simulink model "Pacemaker"  (R2023a)
settings: Solver=FixedStepAuto  StartTime=0.0  StopTime=inf  FixedStep=0.001  RelTol=1e-3  EnableMultiTasking=on
undefined symbols (not defined in the file): D0, D1, D10, D11, D12, D13, D2, D3, D4, D5, D6, D7, D8, D9, PTA0, PTA1, PTA2, PTB23, PTB9, PTC16, PTC17, PTC2, PTC3, PTC4, PTD0, PTD1, PTD2, PTD3
libraries: frdmk64flib x15
settings Model: ExtModeTrigDuration=5  Creator=tstic  LastModifiedBy=nehac
settings OptimizationCC: EnhancedBackFolding=on  PassReuseOutputArgsAs=Individual arguments  ZeroExternalMemoryAtStartup=off  ZeroInternalMemoryAtStartup=off  MaxStackSize=64  OptimizeBlockOrder=speed  DifferentSizesBufferReuse=on  OptimizationCustomize=off  EfficientTunableParamExpr=on
settings DebuggingCC: ParameterTunabilityLossMsg=error
settings HardwareCC: ProdBitPerPointer=32  ProdBitPerSizeT=32  ProdBitPerPtrDiffT=32  ProdLargestAtomicInteger=Long  ProdLargestAtomicFloat=Double  ProdWordSize=32  ProdHWDeviceType=ARM Compatible->ARM Cortex
settings SFSimCC: MATLABDynamicMemAlloc=off
settings RTWCC: Description=Embedded Coder  SystemTargetFile=ert.tlc  HardwareBoard=NXP FRDM-K64F  TLCOptions="-aInlineSetEventsForThisBaseRateFcn=TLC_FALSE -aSuppressMultiTaskScheduler=TLC_FALSE  -aRateBasedStepFcn=0"  TemplateMakefile=ert_default_tmf  Toolchain=GNU Tools for ARM Embedded Processors
settings CodeAppCC: ForceParamTrailComments=on  IgnoreCustomStorageClasses=off  OperatorAnnotations=on  SimulinkDataObjDesc=on  SFDataObjDesc=on  InsertBlockDesc=on
settings ERTTargetCC: ExtModeTransport=4  ExtModeMexFile=sendToCommService

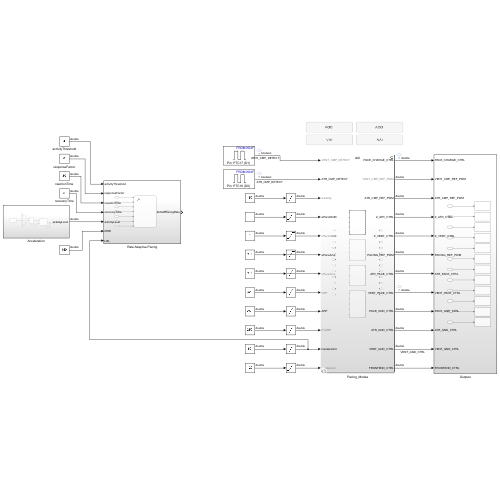
[thumbnail: Simulink's stored preview of the top-level diagram]
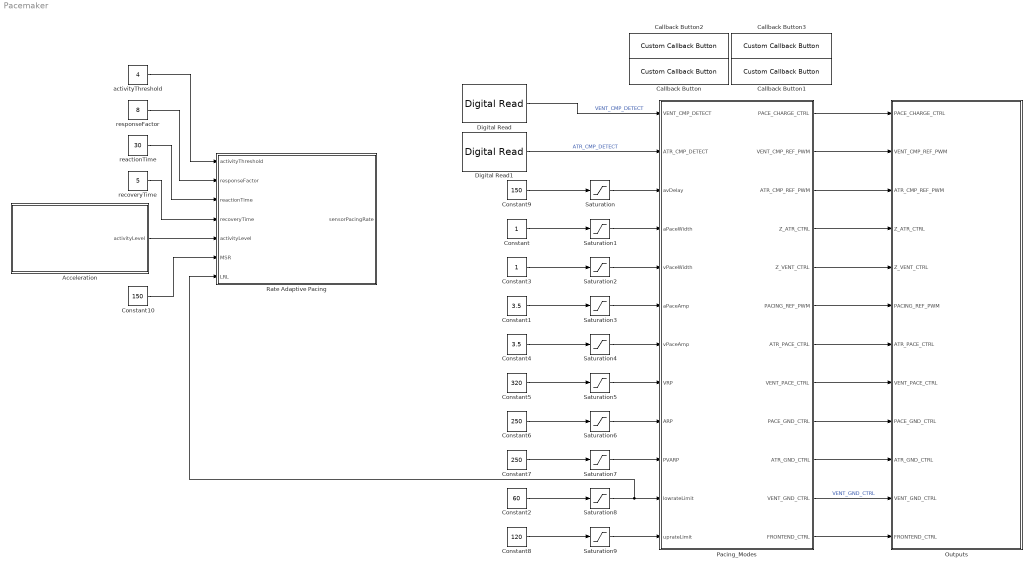
== system Pacemaker ==
  Acceleration : Subsystem
  Callback Button : CustomCallbackButton  Configuration="{\"components\":[{\"name\":\"BackgroundImageComponent\",\"settings\":{\"image\":{\"size\":[0,0],\"src\":\"default\",\"srcOrientation\":\"Right\"},\"position\":[0,0,1,1]}},{\"name\":\"ButtonStateComponent\",\"settings\":{\"buttonType\":\"momentary\",\"clickFcn\":\"myVCV = PacingMode.VVI;\",\"onValue\":1,\"position\":[0,0,1,1],\"pressDelay\":\"500\",\"pressFcn\":\"\",\"repeatInterval\":\"0\",\"states\":[{\"horizontalAlignment\":\"center\",\"image\":{\"position\":[0,0,1,1],\"size\":[1,1],\"src\":\"default\",\"srcOrientation\":\"Right\"},\"label\":{\"color\":[0.01176470588,0.01176470588,0.01176470588,1],\"icon\":{\"size\":[0,0],\"src\":\"default\",\"srcOrientation\":\"Right\"},\"iconPlacement\":\"left\",\"opacity\":1,\"show\":true,\"text\":{\"content\":\"VVI\",\"font\":\"Helvetica\",\"fontSize\":24}},\"labelOffset\":[0,0],\"verticalAlignment\":\"middle\"},{\"horizontalAlignment\":\"center\",\"image\":{\"position\":[0,0,1,1],\"size\":[1,1],\"src\":\"default\",\"srcOrientation\":\"Right\"},\"label\":{\"color\":[0.01176470588,0.01176470588,0.01176470588,1],\"icon\":{\"size\":[0,0],\"src\":\"default\",\"srcOrientation\":\"Right\"},\"iconPlacement\":\"left\",\"opacity\":1,\"show\":true,\"text\":{\"content\":\"VVI\",\"font\":\"Helvetica\",\"fontSize\":24}},\"labelOffset\":[0,0],\"verticalAlignment\":\"middle\"},{\"horizontalAlignment\":\"center\",\"image\":{\"position\":[0,0,1,1],\"size\":[1,1],\"src\":\"default\",\"srcOrientation\":\"Right\"},\"label\":{\"color\":[0.01176470588,0.01176470588,0.01176470588,1],\"icon\":{\"size\":[0,0],\"src\":\"default\",\"srcOrientation\":\"Right\"},\"iconPlacement\":\"left\",\"opacity\":1,\"show\":true,\"text\":{\"content\":\"VVI\",\"font\":\"Helvetica\",\"fontSize\":24}},\"labelOffset\":[0,0],\"verticalAlignment\":\"middle\"},{\"horizontalAlignment\":\"center\",\"image\":{\"position\":[0,0,1,1],\"size\":[1,1],\"src\":\"default\",\"srcOrientation\":\"Right\"},\"label\":{\"color\":[0.01176470588,0.01176470588,0.01176470588,1],\"icon\":{\"size\":[0,0],\"src\":\"default\",\"srcOrientation\":\"Right\"},\"iconPlacement\":\"left\",\"opacity\":1,\"show\":true,\"text\":{\"content\":\"VVI\",\"font\":\"Helvetica\",\"fontSize\":24}},\"labelOffset\":[0,0],\"verticalAlignment\":\"middle\"}]}},{\"name\":\"ForegroundImageComponent\",\"settings\":{\"image\":{\"size\":[0,0],\"src\":\"default\",\"srcOrientation\":\"Right\"},\"isForeground\":1,\"position\":[0,0,1,1]}}],\"settings\":{\"BindingType\":\"standalone\",\"backgroundColor\":[244,244,244,1],\"backgroundOffset\":0.2,\"backgroundOpacity\":1,\"fixedAspectRatio\":\"off\",\"foregroundColor\":[0.01176470588,0.01176470588,0.01176470588,1],\"migratedFromLegacy\":true,\"useBackgroundColor\":true,\"variant\":\"callback\",\"version\":\"R2023a\"},\"type\":\"Button\"}"  CustomBackgroundColor="{\"color\":[0.9568627450980393,0.9568627450980393,0.9568627450980393],\"show\":true}"
  Callback Button1 : CustomCallbackButton  Configuration="{\"components\":[{\"name\":\"BackgroundImageComponent\",\"settings\":{\"image\":{\"size\":[0,0],\"src\":\"default\",\"srcOrientation\":\"Right\"},\"position\":[0,0,1,1]}},{\"name\":\"ButtonStateComponent\",\"settings\":{\"buttonType\":\"momentary\",\"clickFcn\":\"myVCV = PacingMode.AAI;\",\"onValue\":1,\"position\":[0,0,1,1],\"pressDelay\":\"500\",\"pressFcn\":\"\",\"repeatInterval\":\"0\",\"states\":[{\"horizontalAlignment\":\"center\",\"image\":{\"position\":[0,0,1,1],\"size\":[1,1],\"src\":\"default\",\"srcOrientation\":\"Right\"},\"label\":{\"color\":[0.01176470588,0.01176470588,0.01176470588,1],\"icon\":{\"size\":[0,0],\"src\":\"default\",\"srcOrientation\":\"Right\"},\"iconPlacement\":\"left\",\"opacity\":1,\"show\":true,\"text\":{\"content\":\"AAI\",\"font\":\"Helvetica\",\"fontSize\":27}},\"labelOffset\":[0,0],\"verticalAlignment\":\"middle\"},{\"horizontalAlignment\":\"center\",\"image\":{\"position\":[0,0,1,1],\"size\":[1,1],\"src\":\"default\",\"srcOrientation\":\"Right\"},\"label\":{\"color\":[0.01176470588,0.01176470588,0.01176470588,1],\"icon\":{\"size\":[0,0],\"src\":\"default\",\"srcOrientation\":\"Right\"},\"iconPlacement\":\"left\",\"opacity\":1,\"show\":true,\"text\":{\"content\":\"AAI\",\"font\":\"Helvetica\",\"fontSize\":27}},\"labelOffset\":[0,0],\"verticalAlignment\":\"middle\"},{\"horizontalAlignment\":\"center\",\"image\":{\"position\":[0,0,1,1],\"size\":[1,1],\"src\":\"default\",\"srcOrientation\":\"Right\"},\"label\":{\"color\":[0.01176470588,0.01176470588,0.01176470588,1],\"icon\":{\"size\":[0,0],\"src\":\"default\",\"srcOrientation\":\"Right\"},\"iconPlacement\":\"left\",\"opacity\":1,\"show\":true,\"text\":{\"content\":\"AAI\",\"font\":\"Helvetica\",\"fontSize\":27}},\"labelOffset\":[0,0],\"verticalAlignment\":\"middle\"},{\"horizontalAlignment\":\"center\",\"image\":{\"position\":[0,0,1,1],\"size\":[1,1],\"src\":\"default\",\"srcOrientation\":\"Right\"},\"label\":{\"color\":[0.01176470588,0.01176470588,0.01176470588,1],\"icon\":{\"size\":[0,0],\"src\":\"default\",\"srcOrientation\":\"Right\"},\"iconPlacement\":\"left\",\"opacity\":1,\"show\":true,\"text\":{\"content\":\"AAI\",\"font\":\"Helvetica\",\"fontSize\":27}},\"labelOffset\":[0,0],\"verticalAlignment\":\"middle\"}]}},{\"name\":\"ForegroundImageComponent\",\"settings\":{\"image\":{\"size\":[0,0],\"src\":\"default\",\"srcOrientation\":\"Right\"},\"isForeground\":1,\"position\":[0,0,1,1]}}],\"settings\":{\"BindingType\":\"standalone\",\"backgroundColor\":[244,244,244,1],\"backgroundOffset\":0.2,\"backgroundOpacity\":1,\"fixedAspectRatio\":\"off\",\"foregroundColor\":[0.01176470588,0.01176470588,0.01176470588,1],\"migratedFromLegacy\":true,\"useBackgroundColor\":true,\"variant\":\"callback\",\"version\":\"R2023a\"},\"type\":\"Button\"}"  CustomBackgroundColor="{\"color\":[0.9568627450980393,0.9568627450980393,0.9568627450980393],\"show\":true}"
  Callback Button2 : CustomCallbackButton  Configuration="{\"components\":[{\"name\":\"BackgroundImageComponent\",\"settings\":{\"image\":{\"size\":[0,0],\"src\":\"default\",\"srcOrientation\":\"Right\"},\"position\":[0,0,1,1]}},{\"name\":\"ButtonStateComponent\",\"settings\":{\"buttonType\":\"momentary\",\"clickFcn\":\"myVCV = PacingMode.VOO;\",\"onValue\":1,\"position\":[0,0,1,1],\"pressDelay\":\"500\",\"pressFcn\":\"\",\"repeatInterval\":\"0\",\"states\":[{\"horizontalAlignment\":\"center\",\"image\":{\"position\":[0,0,1,1],\"size\":[1,1],\"src\":\"default\",\"srcOrientation\":\"Right\"},\"label\":{\"color\":[0.01176470588,0.01176470588,0.01176470588,1],\"icon\":{\"size\":[0,0],\"src\":\"default\",\"srcOrientation\":\"Right\"},\"iconPlacement\":\"left\",\"opacity\":1,\"show\":true,\"text\":{\"content\":\"VOO\",\"font\":\"Helvetica\",\"fontSize\":27}},\"labelOffset\":[0,0],\"verticalAlignment\":\"middle\"},{\"horizontalAlignment\":\"center\",\"image\":{\"position\":[0,0,1,1],\"size\":[1,1],\"src\":\"default\",\"srcOrientation\":\"Right\"},\"label\":{\"color\":[0.01176470588,0.01176470588,0.01176470588,1],\"icon\":{\"size\":[0,0],\"src\":\"default\",\"srcOrientation\":\"Right\"},\"iconPlacement\":\"left\",\"opacity\":1,\"show\":true,\"text\":{\"content\":\"VOO\",\"font\":\"Helvetica\",\"fontSize\":27}},\"labelOffset\":[0,0],\"verticalAlignment\":\"middle\"},{\"horizontalAlignment\":\"center\",\"image\":{\"position\":[0,0,1,1],\"size\":[1,1],\"src\":\"default\",\"srcOrientation\":\"Right\"},\"label\":{\"color\":[0.01176470588,0.01176470588,0.01176470588,1],\"icon\":{\"size\":[0,0],\"src\":\"default\",\"srcOrientation\":\"Right\"},\"iconPlacement\":\"left\",\"opacity\":1,\"show\":true,\"text\":{\"content\":\"VOO\",\"font\":\"Helvetica\",\"fontSize\":27}},\"labelOffset\":[0,0],\"verticalAlignment\":\"middle\"},{\"horizontalAlignment\":\"center\",\"image\":{\"position\":[0,0,1,1],\"size\":[1,1],\"src\":\"default\",\"srcOrientation\":\"Right\"},\"label\":{\"color\":[0.01176470588,0.01176470588,0.01176470588,1],\"icon\":{\"size\":[0,0],\"src\":\"default\",\"srcOrientation\":\"Right\"},\"iconPlacement\":\"left\",\"opacity\":1,\"show\":true,\"text\":{\"content\":\"VOO\",\"font\":\"Helvetica\",\"fontSize\":27}},\"labelOffset\":[0,0],\"verticalAlignment\":\"middle\"}]}},{\"name\":\"ForegroundImageComponent\",\"settings\":{\"image\":{\"size\":[0,0],\"src\":\"default\",\"srcOrientation\":\"Right\"},\"isForeground\":1,\"position\":[0,0,1,1]}}],\"settings\":{\"BindingType\":\"standalone\",\"backgroundColor\":[244,244,244,1],\"backgroundOffset\":0.2,\"backgroundOpacity\":1,\"fixedAspectRatio\":\"off\",\"foregroundColor\":[0.01176470588,0.01176470588,0.01176470588,1],\"migratedFromLegacy\":true,\"useBackgroundColor\":true,\"variant\":\"callback\",\"version\":\"R2023a\"},\"type\":\"Button\"}"  CustomBackgroundColor="{\"color\":[0.9568627450980393,0.9568627450980393,0.9568627450980393],\"show\":true}"
  Callback Button3 : CustomCallbackButton  Configuration="{\"components\":[{\"name\":\"BackgroundImageComponent\",\"settings\":{\"image\":{\"size\":[0,0],\"src\":\"default\",\"srcOrientation\":\"Right\"},\"position\":[0,0,1,1]}},{\"name\":\"ButtonStateComponent\",\"settings\":{\"buttonType\":\"momentary\",\"clickFcn\":\"myVCV = PacingMode.AOO;\",\"onValue\":1,\"position\":[0,0,1,1],\"pressDelay\":\"500\",\"pressFcn\":\"\",\"repeatInterval\":\"0\",\"states\":[{\"horizontalAlignment\":\"center\",\"image\":{\"position\":[0,0,1,1],\"size\":[1,1],\"src\":\"default\",\"srcOrientation\":\"Right\"},\"label\":{\"color\":[0.01176470588,0.01176470588,0.01176470588,1],\"icon\":{\"size\":[0,0],\"src\":\"default\",\"srcOrientation\":\"Right\"},\"iconPlacement\":\"left\",\"opacity\":1,\"show\":true,\"text\":{\"content\":\"AOO\",\"font\":\"Helvetica\",\"fontSize\":27}},\"labelOffset\":[0,0],\"verticalAlignment\":\"middle\"},{\"horizontalAlignment\":\"center\",\"image\":{\"position\":[0,0,1,1],\"size\":[1,1],\"src\":\"default\",\"srcOrientation\":\"Right\"},\"label\":{\"color\":[0.01176470588,0.01176470588,0.01176470588,1],\"icon\":{\"size\":[0,0],\"src\":\"default\",\"srcOrientation\":\"Right\"},\"iconPlacement\":\"left\",\"opacity\":1,\"show\":true,\"text\":{\"content\":\"AOO\",\"font\":\"Helvetica\",\"fontSize\":27}},\"labelOffset\":[0,0],\"verticalAlignment\":\"middle\"},{\"horizontalAlignment\":\"center\",\"image\":{\"position\":[0,0,1,1],\"size\":[1,1],\"src\":\"default\",\"srcOrientation\":\"Right\"},\"label\":{\"color\":[0.01176470588,0.01176470588,0.01176470588,1],\"icon\":{\"size\":[0,0],\"src\":\"default\",\"srcOrientation\":\"Right\"},\"iconPlacement\":\"left\",\"opacity\":1,\"show\":true,\"text\":{\"content\":\"AOO\",\"font\":\"Helvetica\",\"fontSize\":27}},\"labelOffset\":[0,0],\"verticalAlignment\":\"middle\"},{\"horizontalAlignment\":\"center\",\"image\":{\"position\":[0,0,1,1],\"size\":[1,1],\"src\":\"default\",\"srcOrientation\":\"Right\"},\"label\":{\"color\":[0.01176470588,0.01176470588,0.01176470588,1],\"icon\":{\"size\":[0,0],\"src\":\"default\",\"srcOrientation\":\"Right\"},\"iconPlacement\":\"left\",\"opacity\":1,\"show\":true,\"text\":{\"content\":\"AOO\",\"font\":\"Helvetica\",\"fontSize\":27}},\"labelOffset\":[0,0],\"verticalAlignment\":\"middle\"}]}},{\"name\":\"ForegroundImageComponent\",\"settings\":{\"image\":{\"size\":[0,0],\"src\":\"default\",\"srcOrientation\":\"Right\"},\"isForeground\":1,\"position\":[0,0,1,1]}}],\"settings\":{\"BindingType\":\"standalone\",\"backgroundColor\":[244,244,244,1],\"backgroundOffset\":0.2,\"backgroundOpacity\":1,\"fixedAspectRatio\":\"off\",\"foregroundColor\":[0.01176470588,0.01176470588,0.01176470588,1],\"migratedFromLegacy\":true,\"useBackgroundColor\":true,\"variant\":\"callback\",\"version\":\"R2023a\"},\"type\":\"Button\"}"  CustomBackgroundColor="{\"color\":[0.9568627450980393,0.9568627450980393,0.9568627450980393],\"show\":true}"
  Constant : Constant
  Constant1 : Constant  Value=3.5
  Constant10 : Constant  Value=150
  Constant2 : Constant  Value=60
  Constant3 : Constant
  Constant4 : Constant  Value=3.5
  Constant5 : Constant  Value=320
  Constant6 : Constant  Value=250
  Constant7 : Constant  Value=250
  Constant8 : Constant  Value=120
  Constant9 : Constant  Value=150
  Digital Read : frdmk64flib/Digital Read  Whichpin=PTC17 (D1)  SampleTime=0.001
  Digital Read1 : frdmk64flib/Digital Read  Whichpin=PTC16 (D0)  SampleTime=0.001
  Outputs : Subsystem
  Pacing_Modes : Subsystem  Variant=on  VariantChoicesEnumeration=PacingMode  VariantControlVariable=myVCV
  Rate Adaptive Pacing : Subsystem
  Saturation : Saturate  UpperLimit=300  LowerLimit=70
  Saturation1 : Saturate  UpperLimit=1.9  LowerLimit=0.1
  Saturation2 : Saturate  UpperLimit=1.9  LowerLimit=0.1
  Saturation3 : Saturate  UpperLimit=5  LowerLimit=0.5
  Saturation4 : Saturate  UpperLimit=5  LowerLimit=0.5
  Saturation5 : Saturate  UpperLimit=500  LowerLimit=150
  Saturation6 : Saturate  UpperLimit=500  LowerLimit=150
  Saturation7 : Saturate  UpperLimit=500  LowerLimit=150
  Saturation8 : Saturate  UpperLimit=175  LowerLimit=30
  Saturation9 : Saturate  UpperLimit=175  LowerLimit=50
  activityThreshold : Constant  Value=4
  reactionTime : Constant  Value=30
  recoveryTime : Constant  Value=5
  responseFactor : Constant  Value=8
  wires:
  Digital Read1/1 -> Pacing_Modes/2(ATR_CMP_DETECT)  "ATR_CMP_DETECT"
  Digital Read/1 -> Pacing_Modes/1(VENT_CMP_DETECT)  "VENT_CMP_DETECT"
  Constant/1 -> Saturation1/1
  Constant1/1 -> Saturation3/1
  Constant2/1 -> Saturation8/1
  Constant3/1 -> Saturation2/1
  Constant4/1 -> Saturation4/1
  Constant6/1 -> Saturation6/1
  Constant5/1 -> Saturation5/1
  Constant7/1 -> Saturation7/1
  Constant8/1 -> Saturation9/1
  Constant9/1 -> Saturation/1
  Saturation/1 -> Pacing_Modes/3(avDelay)
  Saturation1/1 -> Pacing_Modes/4(aPaceWidth)
  Saturation2/1 -> Pacing_Modes/5(vPaceWidth)
  Saturation3/1 -> Pacing_Modes/6(aPaceAmp)
  Saturation4/1 -> Pacing_Modes/7(vPaceAmp)
  Saturation5/1 -> Pacing_Modes/8(VRP)
  Saturation6/1 -> Pacing_Modes/9(ARP)
  Saturation7/1 -> Pacing_Modes/10(PVARP)
  Saturation8/1 -> Rate Adaptive Pacing/7(LRL), Pacing_Modes/11(lowrateLimit)
  Saturation9/1 -> Pacing_Modes/12(uprateLimit)
  Acceleration/1(activityLevel) -> Rate Adaptive Pacing/5(activityLevel)
  Constant10/1 -> Rate Adaptive Pacing/6(MSR)
  activityThreshold/1 -> Rate Adaptive Pacing/1(activityThreshold)
  responseFactor/1 -> Rate Adaptive Pacing/2(responseFactor)
  reactionTime/1 -> Rate Adaptive Pacing/3(reactionTime)
  recoveryTime/1 -> Rate Adaptive Pacing/4(recoveryTime)
  Pacing_Modes/1(PACE_CHARGE_CTRL) -> Outputs/1(PACE_CHARGE_CTRL)
  Pacing_Modes/2(VENT_CMP_REF_PWM) -> Outputs/2(VENT_CMP_REF_PWM)
  Pacing_Modes/3(ATR_CMP_REF_PWM) -> Outputs/3(ATR_CMP_REF_PWM)
  Pacing_Modes/4(Z_ATR_CTRL) -> Outputs/4(Z_ATR_CTRL)
  Pacing_Modes/5(Z_VENT_CTRL) -> Outputs/5(Z_VENT_CTRL)
  Pacing_Modes/6(PACING_REF_PWM) -> Outputs/6(PACING_REF_PWM)
  Pacing_Modes/7(ATR_PACE_CTRL) -> Outputs/7(ATR_PACE_CTRL)
  Pacing_Modes/8(VENT_PACE_CTRL) -> Outputs/8(VENT_PACE_CTRL)
  Pacing_Modes/9(PACE_GND_CTRL) -> Outputs/9(PACE_GND_CTRL)
  Pacing_Modes/10(ATR_GND_CTRL) -> Outputs/10(ATR_GND_CTRL)
  Pacing_Modes/11(VENT_GND_CTRL) -> Outputs/11(VENT_GND_CTRL)  "VENT_GND_CTRL"
  Pacing_Modes/12(FRONTEND_CTRL) -> Outputs/12(FRONTEND_CTRL)

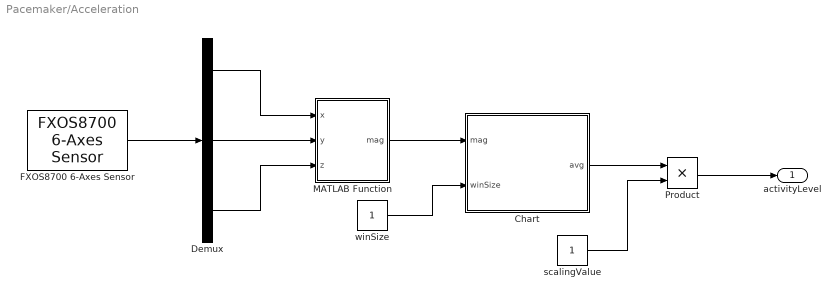
== system Pacemaker/Acceleration ==
  Chart : Stateflow chart  TreatAsAtomicUnit=on
  Demux : Demux  Outputs=3
  FXOS8700 6-Axes Sensor : frdmk64flib/FXOS8700 6-Axes Sensor  Activesensor=Accelerometer only  ODR=800Hz  HybridODR=400Hz  Accelfullrange=-4g to +4g  SampleTime=0.01
  MATLAB Function : MATLAB Function  TreatAsAtomicUnit=on
  Product : Product
  scalingValue : Constant
  winSize : Constant
  activityLevel : Outport
  wires:
  FXOS8700 6-Axes Sensor/1 -> Demux/1
  winSize/1 -> Chart/2(winSize)
  Demux/1 -> MATLAB Function/1(x)
  Demux/2 -> MATLAB Function/2(y)
  Demux/3 -> MATLAB Function/3(z)
  MATLAB Function/1(mag) -> Chart/1(mag)
  Chart/1(avg) -> Product/1
  scalingValue/1 -> Product/2
  Product/1 -> activityLevel/1

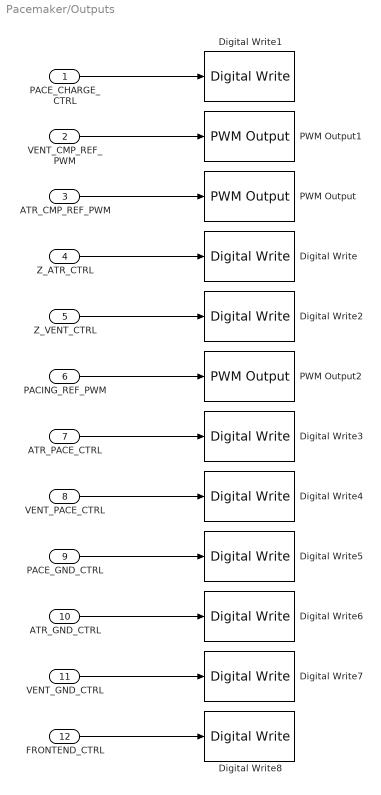
== system Pacemaker/Outputs ==
  PACE_CHARGE_CTRL : Inport
  VENT_CMP_REF_PWM : Inport  Port=2
  ATR_CMP_REF_PWM : Inport  Port=3
  Z_ATR_CTRL : Inport  Port=4
  Z_VENT_CTRL : Inport  Port=5
  PACING_REF_PWM : Inport  Port=6
  ATR_PACE_CTRL : Inport  Port=7
  VENT_PACE_CTRL : Inport  Port=8
  PACE_GND_CTRL : Inport  Port=9
  ATR_GND_CTRL : Inport  Port=10
  VENT_GND_CTRL : Inport  Port=11
  FRONTEND_CTRL : Inport  Port=12
  Digital Write : frdmk64flib/Digital Write  Whichpin=PTB23 (D4)
  Digital Write1 : frdmk64flib/Digital Write  Whichpin=PTB9 (D2)
  Digital Write2 : frdmk64flib/Digital Write  Whichpin=PTC3 (D7)
  Digital Write3 : frdmk64flib/Digital Write  Whichpin=PTA0 (D8)
  Digital Write4 : frdmk64flib/Digital Write  Whichpin=PTC4 (D9)
  Digital Write5 : frdmk64flib/Digital Write  Whichpin=PTD0 (D10)
  Digital Write6 : frdmk64flib/Digital Write  Whichpin=PTD2 (D11)
  Digital Write7 : frdmk64flib/Digital Write  Whichpin=PTD3 (D12)
  Digital Write8 : frdmk64flib/Digital Write  Whichpin=PTD1 (D13)
  PWM Output : frdmk64flib/PWM Output  Whichpin=PTC2 (D6)  InitialFrequency=2000  InitialDutyCycle=0
  PWM Output1 : frdmk64flib/PWM Output  Whichpin=PTA1 (D3)  InitialFrequency=2000  InitialDutyCycle=0
  PWM Output2 : frdmk64flib/PWM Output  Whichpin=PTA2 (D5)  InitialFrequency=2000  InitialDutyCycle=0
  wires:
  Z_ATR_CTRL/1 -> Digital Write/1
  PACING_REF_PWM/1 -> PWM Output2/1
  ATR_PACE_CTRL/1 -> Digital Write3/1
  VENT_CMP_REF_PWM/1 -> PWM Output1/1
  PACE_CHARGE_CTRL/1 -> Digital Write1/1
  VENT_PACE_CTRL/1 -> Digital Write4/1
  VENT_GND_CTRL/1 -> Digital Write7/1
  ATR_CMP_REF_PWM/1 -> PWM Output/1
  PACE_GND_CTRL/1 -> Digital Write5/1
  FRONTEND_CTRL/1 -> Digital Write8/1
  Z_VENT_CTRL/1 -> Digital Write2/1
  ATR_GND_CTRL/1 -> Digital Write6/1

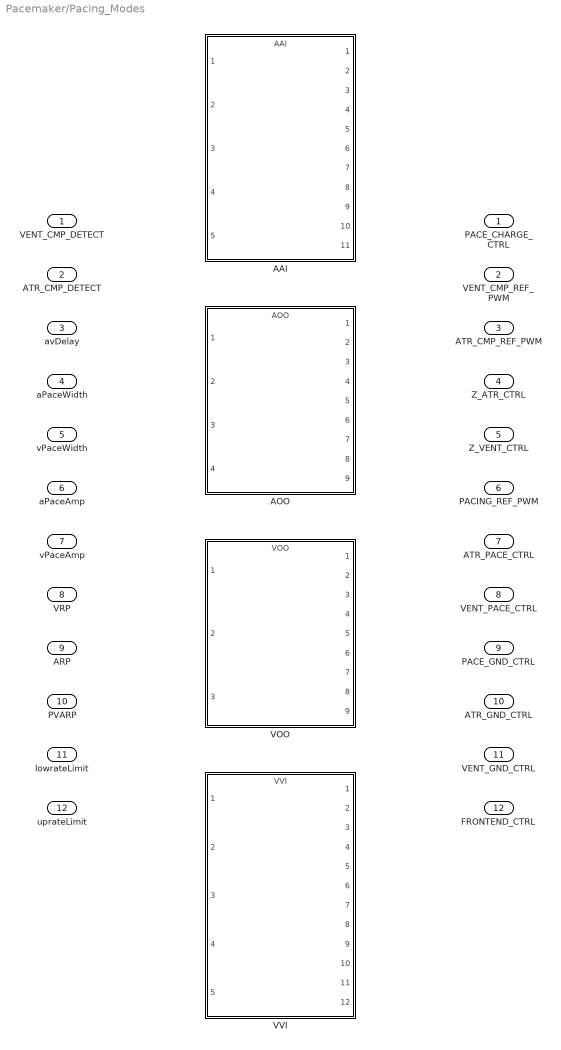
== system Pacemaker/Pacing_Modes ==
  VENT_CMP_DETECT : Inport
  ATR_CMP_DETECT : Inport  Port=2
  avDelay : Inport  Port=3
  aPaceWidth : Inport  Port=4
  vPaceWidth : Inport  Port=5
  aPaceAmp : Inport  Port=6
  vPaceAmp : Inport  Port=7
  VRP : Inport  Port=8
  ARP : Inport  Port=9
  PVARP : Inport  Port=10
  lowrateLimit : Inport  Port=11
  uprateLimit : Inport  Port=12
  AAI : ModelReference  ModelNameDialog=AAI  SimulationMode=Normal  VariantControl=myVCV == PacingMode.AAI  ModelReferenceVersion=1.74
  AOO : ModelReference  ModelNameDialog=AOO  SimulationMode=Normal  VariantControl=myVCV == PacingMode.AOO  ModelReferenceVersion=1.28
  VOO : ModelReference  ModelNameDialog=VOO  SimulationMode=Normal  VariantControl=myVCV == PacingMode.VOO  ModelReferenceVersion=1.13
  VVI : ModelReference  ModelNameDialog=VVI.slx  SimulationMode=Normal  VariantControl=myVCV == PacingMode.VVI  ModelReferenceVersion=1.46
  PACE_CHARGE_CTRL : Outport
  VENT_CMP_REF_PWM : Outport  Port=2
  ATR_CMP_REF_PWM : Outport  Port=3
  Z_ATR_CTRL : Outport  Port=4
  Z_VENT_CTRL : Outport  Port=5
  PACING_REF_PWM : Outport  Port=6
  ATR_PACE_CTRL : Outport  Port=7
  VENT_PACE_CTRL : Outport  Port=8
  PACE_GND_CTRL : Outport  Port=9
  ATR_GND_CTRL : Outport  Port=10
  VENT_GND_CTRL : Outport  Port=11
  FRONTEND_CTRL : Outport  Port=12

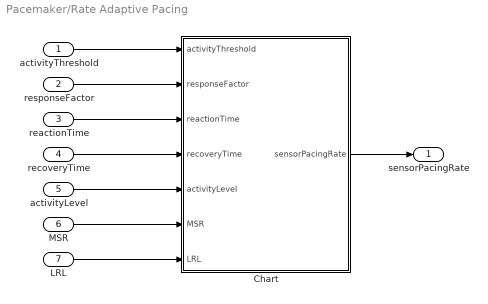
== system Pacemaker/Rate Adaptive Pacing ==
  activityThreshold : Inport
  responseFactor : Inport  Port=2
  reactionTime : Inport  Port=3
  recoveryTime : Inport  Port=4
  activityLevel : Inport  Port=5
  MSR : Inport  Port=6
  LRL : Inport  Port=7
  Chart : Stateflow chart  TreatAsAtomicUnit=on
  sensorPacingRate : Outport
  wires:
  activityThreshold/1 -> Chart/1(activityThreshold)
  responseFactor/1 -> Chart/2(responseFactor)
  reactionTime/1 -> Chart/3(reactionTime)
  recoveryTime/1 -> Chart/4(recoveryTime)
  activityLevel/1 -> Chart/5(activityLevel)
  MSR/1 -> Chart/6(MSR)
  LRL/1 -> Chart/7(LRL)
  Chart/1(sensorPacingRate) -> sensorPacingRate/1

== matlab function Pacemaker/Acceleration/MATLAB Function ==
  data: x input; mag output; y input; z input
function mag = fcn(x, y, z)

mag = (x^2 + y^2 + z^2)^0.5;

== stateflow chart Pacemaker/Acceleration/Chart ==
  state Collect
    entry:
    sum = sum + mag;
    collected = collected + 1;
  state Smooth
    entry:
    avg = sum / winSize;
  (default) -> Collect : {collected = 0; sum = 0}
  Collect -> (junction 17)
  (junction 17) -> Smooth [order 1] : [collected == winSize]
  (junction 17) -> Collect [order 2] : [collected < winSize]
  Smooth -> Collect : {collected = 0; sum = 0;}
  data: mag input; winSize input; collected local; avg output; sum local

== stateflow chart Pacemaker/Rate Adaptive Pacing/Chart ==
  state DPR
    entry:
    %% ?? what do you use responseFactor for??
    scale = (responseFactor/16)*((MSR - activityThreshold)/MSR);
    desiredPacingRate = scale*(activityLevel - activityThreshold) + LRL;
    if (desiredPacingRate < LRL)
    desiredPacingRate = LRL;
    end
    if (desiredPacingRate > MSR)
    desiredPacingRate = MSR;
    end
  state SPR
    entry:
    reactionStep = (MSR - LRL)/(reactionTime*1000);
    recoveryStep = (MSR - LRL)/(recoveryTime*60000);
    if currentPacingRate < desiredPacingRate
    sensorPacingRate = currentPacingRate + 10*reactionStep;
    end
    if currentPacingRate > desiredPacingRate
    sensorPacingRate = currentPacingRate - 10*recoveryStep;
    end
  SPR -> DPR : [after(10,msec)]{currentPacingRate = sensorPacingRate;}
  (default) -> DPR : {currentPacingRate = LRL; sensorPacingRate = LRL}
  DPR -> SPR
  data: activityThreshold input; responseFactor input; reactionTime input; recoveryTime input; activityLevel input; MSR input; LRL input; sensorPacingRate output; desiredPacingRate local; currentPacingRate local; reactionStep local; recoveryStep local; scale local
